simulink model "Fd_2Hz"  (R2017b)
settings: Solver=VariableStepAuto  StartTime=0.0  StopTime=10.0  RelTol=1e-3  EnableMultiTasking=on
InitFcn:
  | %Digital Modulator
  | M=4;       %MQAM
  | Fs=10e6;   %Symbols Rate
  | Fb=log2(M)*Fs;  %bit rate
  | 
  | %Power Transmitter and Received
  | PT=0.5;      %Transmitter Power in Walts
  | A=1/100;     %channel attennuation
  | PR=A*PT;     %Received Power in Walts
  | 
  | %channel
  | P=[0,-2,-3];    %dB
  | T=[0,15,50]*10^(-9);  %sec
  | fd=2;      %Hz
undefined symbols (not defined in the file): doppler
libraries: commrandsrc3 x1, commchan3 x1, commdigbbndam3 x1
settings Model: Creator=yue  LastModifiedBy=changgang
settings OptimizationCC: LifeSpan=inf
settings DebuggingCC: SFUnexpectedBacktrackingDiag=warning  SFNoUnconditionalDefaultTransitionDiag=warning  SFExecutionAtInitializationDiag=none
settings CodeAppCC: StateflowObjectComments=on
settings GRTTargetCC: TargetLangStandard=C89/C90 (ANSI)  GeneratePreprocessorConditionals=Disable all
settings ConfigComp: CovMetricSettings=dw  CovHtmlReporting=on  CovSaveCumulativeToWorkspaceVar=on  CovSaveSingleToWorkspaceVar=on  CovExternalEMLEnable=off

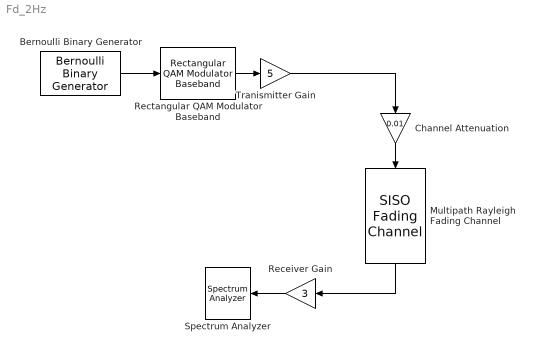
== system Fd_2Hz ==
  Bernoulli Binary Generator : commrandsrc3/Bernoulli Binary Generator  ProbabilityOfZero=0.5  SeedSource=Parameter  Seed=61  SampleTime=1/Fb  SamplesPerFrame=log2(M)  OutputDataType=single  SimulateUsing=Interpreted execution
  Channel Attenuation : Gain  Gain=0.01
  Multipath Rayleigh Fading Channel : commchan3/SISO Fading Channel  PathDelays=T  AveragePathGains=P  NormalizePathGains=on  FadingDistribution=Rayleigh  KFactor=3  DirectPathDopplerShift=0  DirectPathInitialPhase=0  MaximumDopplerShift=fd  DopplerSpectrum=doppler('Jakes')  RandomStream=mt19937ar with seed  RandomNumGenerator=shr3cong  Seed=73  PathGainsOutputPort=off  ChannelFilterDelayOutputPort=off  SimulateUsing=Interpreted execution  Visualization=Off  PathsForDopplerDisplay=1  SamplesToDisplay=25%
      settings: SourceProductName=Communications System Toolbox
  Receiver Gain : Gain  Gain=3
  Rectangular QAM Modulator Baseband : commdigbbndam3/Rectangular QAM Modulator Baseband  M=M  InType=Bit  Enc=Gray  Mapping=[0:15]  PowType=Average Power  MinDist=2  AvgPow=1  PeakPow=1  Ph=0  outDtype=double  outWordLen=16  outUDDataType=sfix(16)  outFracLenMode=Best precision  outFracLen=15  outDataTypeStr=double  outLastDataTypeStr=double
  Spectrum Analyzer : SpectrumAnalyzer
  Tranismitter Gain : Gain  Gain=5
  wires:
  Bernoulli Binary Generator/1 -> Rectangular QAM Modulator Baseband/1
  Rectangular QAM Modulator Baseband/1 -> Tranismitter Gain/1
  Tranismitter Gain/1 -> Channel Attenuation/1
  Channel Attenuation/1 -> Multipath Rayleigh Fading Channel/1
  Multipath Rayleigh Fading Channel/1 -> Receiver Gain/1
  Receiver Gain/1 -> Spectrum Analyzer/1
